simulink model "SAL_sensor"  (R2025b)
settings: Solver=ode4  StartTime=0.0  StopTime=10.0  FixedStep=0.01  RelTol=1e-3
undefined symbols (not defined in the file): s_fov
settings Model: DataDictionary=SAL_sensor_data.sldd  Creator=mauro  LastModifiedBy=mauro

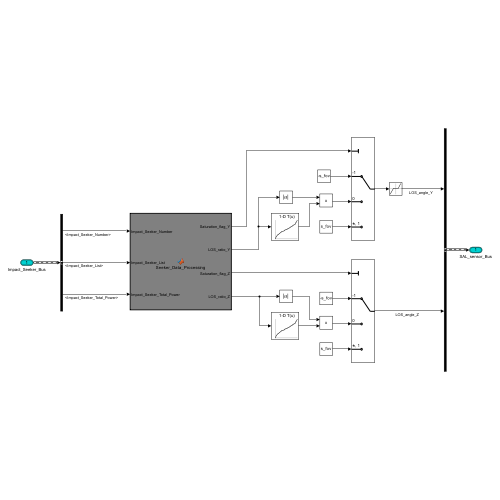
[thumbnail: Simulink's stored preview of the top-level diagram]
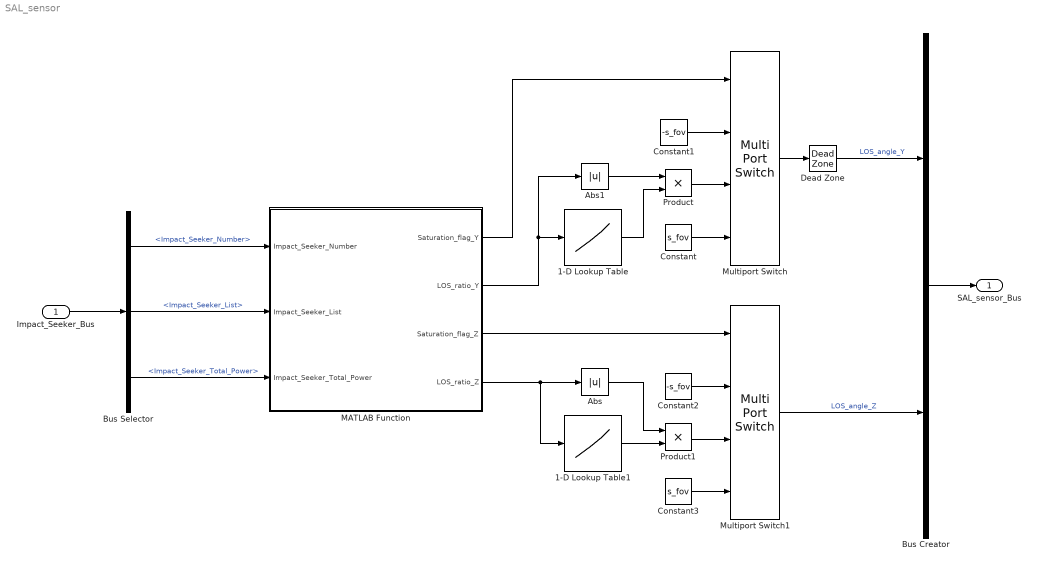
== system SAL_sensor ==
  Impact_Seeker_Bus : Inport  OutDataTypeStr=Bus: Impact_Seeker_Bus  BusOutputAsStruct=on
  1-D Lookup Table : Lookup_n-D  NumberOfTableDimensions=1  BreakpointsForDimension1=[-1.0, -0.9, -0.8, -0.7, -0.6, -0.5, -0.4, -0.3, -0.2, -0.1, 0.0, 0.1, 0.2, 0.3, 0.4, 0.5, 0.6, 0.7, 0.8, 0.9, 1.0]  Table=s_fov*[-1.0, -0.760, -0.600, -0.490, -0.400, -0.320, -0.250, -0.180, -0.120, -0.060, 0.0, 0.060, 0.120, 0.180, 0.250, 0.320, 0.400, 0.490, 0.600, 0.760, 1.0];  ExtrapMethod=Clip  InternalRulePriority=Speed  RndMeth=Simplest
  1-D Lookup Table1 : Lookup_n-D  NumberOfTableDimensions=1  BreakpointsForDimension1=[-1.0, -0.9, -0.8, -0.7, -0.6, -0.5, -0.4, -0.3, -0.2, -0.1, 0.0, 0.1, 0.2, 0.3, 0.4, 0.5, 0.6, 0.7, 0.8, 0.9, 1.0]  Table=s_fov*[-1.0, -0.760, -0.600, -0.490, -0.400, -0.320, -0.250, -0.180, -0.120, -0.060, 0.0, 0.060, 0.120, 0.180, 0.250, 0.320, 0.400, 0.490, 0.600, 0.760, 1.0];  ExtrapMethod=Clip  InternalRulePriority=Speed  RndMeth=Simplest
  Abs : Abs  SaturateOnIntegerOverflow=off
  Abs1 : Abs  SaturateOnIntegerOverflow=off
  Bus Creator : BusCreator  Inputs=2  OutDataTypeStr=Bus: SAL_sensor_Bus  NonVirtualBus=on
  Bus Selector : BusSelector  OutputSignals=Impact_Seeker_Number,Impact_Seeker_List,Impact_Seeker_Total_Power
  Constant : Constant  Value=s_fov
  Constant1 : Constant  Value=-s_fov
  Constant2 : Constant  Value=-s_fov
  Constant3 : Constant  Value=s_fov
  Dead Zone : DeadZone  LowerValue=-1e-4  UpperValue=1e-4
  MATLAB Function : MATLAB Function  TreatAsAtomicUnit=on
  Multiport Switch : MultiPortSwitch  DataPortOrder=Specify indices  DataPortIndices={-1,0,1}  SaturateOnIntegerOverflow=off  InputSameDT=off
  Multiport Switch1 : MultiPortSwitch  DataPortOrder=Specify indices  DataPortIndices={-1,0,1}  SaturateOnIntegerOverflow=off  InputSameDT=off
  Product : Product
  Product1 : Product
  SAL_sensor_Bus : Outport  OutDataTypeStr=Bus: SAL_sensor_Bus  BusOutputAsStruct=on
  wires:
  Impact_Seeker_Bus/1 -> Bus Selector/1
  Bus Creator/1 -> SAL_sensor_Bus/1
  MATLAB Function/1(Saturation_flag_Y) -> Multiport Switch/1
  Constant1/1 -> Multiport Switch/2
  Constant/1 -> Multiport Switch/4
  MATLAB Function/2(LOS_ratio_Y) -> Abs1/1, 1-D Lookup Table/1
  Product/1 -> Multiport Switch/3
  MATLAB Function/3(Saturation_flag_Z) -> Multiport Switch1/1
  Constant2/1 -> Multiport Switch1/2
  Constant3/1 -> Multiport Switch1/4
  Product1/1 -> Multiport Switch1/3
  1-D Lookup Table1/1 -> Product1/2
  MATLAB Function/4(LOS_ratio_Z) -> Abs/1, 1-D Lookup Table1/1
  1-D Lookup Table/1 -> Product/2
  Multiport Switch/1 -> Dead Zone/1
  Bus Selector/2 -> MATLAB Function/2(Impact_Seeker_List)  "<Impact_Seeker_List>"
  Bus Selector/1 -> MATLAB Function/1(Impact_Seeker_Number)  "<Impact_Seeker_Number>"
  Bus Selector/3 -> MATLAB Function/3(Impact_Seeker_Total_Power)  "<Impact_Seeker_Total_Power>"
  Dead Zone/1 -> Bus Creator/1  "LOS_angle_Y"
  Multiport Switch1/1 -> Bus Creator/2  "LOS_angle_Z"
  Abs/1 -> Product1/1
  Abs1/1 -> Product/1

== matlab function SAL_sensor/MATLAB Function ==
  data: Saturation_flag_Y output; Impact_Seeker_Number input; Impact_Seeker_List input; Impact_Seeker_Total_Power input; LOS_ratio_Y output; Saturation_flag_Z output; s_energy_threshold parameter; LOS_ratio_Z output
function [Saturation_flag_Y,LOS_ratio_Y,Saturation_flag_Z,LOS_ratio_Z]= Seeker_Data_Processing(Impact_Seeker_Number,Impact_Seeker_List,Impact_Seeker_Total_Power,s_energy_threshold)

Saturation_flag_Y   = 0;
Saturation_flag_Z   = 0;
LOS_ratio_Y         = 0;
LOS_ratio_Z         = 0;

if Impact_Seeker_Total_Power >= s_energy_threshold

    Q1_power = sum(Impact_Seeker_List(2, 1:Impact_Seeker_Number));
    Q2_power = sum(Impact_Seeker_List(3, 1:Impact_Seeker_Number));
    Q3_power = sum(Impact_Seeker_List(4, 1:Impact_Seeker_Number));
    Q4_power = sum(Impact_Seeker_List(5, 1:Impact_Seeker_Number));

    LOS_ratio_Z = (((Q1_power+Q2_power)-(Q3_power+Q4_power))/Impact_Seeker_Total_Power);
    LOS_ratio_Y = (((Q1_power+Q4_power)-(Q3_power+Q2_power))/Impact_Seeker_Total_Power);

    if LOS_ratio_Y >= 0.999

        Saturation_flag_Y = 1;
    
    end

    if LOS_ratio_Z >= 0.999 

        Saturation_flag_Z = 1;

    end

    if LOS_ratio_Y <= -0.999

        Saturation_flag_Y = -1;
    
    end

    if LOS_ratio_Z <= -0.999 

        Saturation_flag_Z = -1;

    end

end
